simulink model "modelo_control_geoposicion"  (Simulink 7.5)
settings: Solver=ode45  StartTime=0.0  StopTime=10.0  RelTol=1e-3
settings Model: Creator=ARTURO  LastModifiedBy=ARTURO

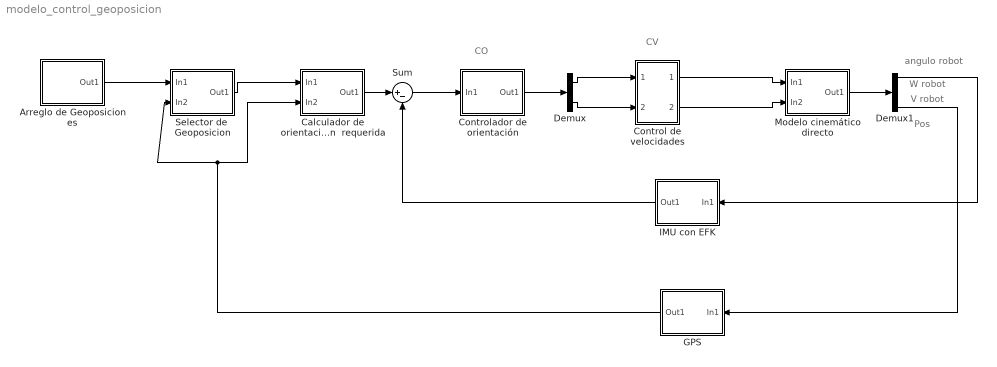
== system modelo_control_geoposicion ==
  note: W robot
  note: V robot
  note: angulo robot
  note: CV
  note: CO
  note: Pos
  Arreglo de Geoposiciones : Subsystem
  Calculador de orientación  requerida : Subsystem
  Control de velocidades : Subsystem
  Controlador de orientación : Subsystem
  Demux : Demux  Outputs=2
  Demux1 : Demux
  GPS : Subsystem
  IMU con EFK : Subsystem
  Modelo cinemático directo : Subsystem
  Selector de  Geoposicion : Subsystem
  Sum : Sum  Inputs=|+-  OutDataType=fixdt(1, 16)  OutScaling=2^0
  wires:
  Demux/1 -> Control de velocidades/1(In1)
  Demux/2 -> Control de velocidades/2(In2)
  Modelo cinemático directo/1(Out1) -> Demux1/1
  Control de velocidades/1(Out1) -> Modelo cinemático directo/1(In1)
  Control de velocidades/2(Out2) -> Modelo cinemático directo/2(In2)
  Calculador de orientación  requerida/1(Out1) -> Sum/1
  Sum/1 -> Controlador de orientación/1(In1)
  Controlador de orientación/1(Out1) -> Demux/1
  Demux1/1 -> IMU con EFK/1(In1)
  IMU con EFK/1(Out1) -> Sum/2
  Demux1/4 -> GPS/1(In1)
  Selector de  Geoposicion/1(Out1) -> Calculador de orientación  requerida/1(In1)
  GPS/1(Out1) -> Calculador de orientación  requerida/2(In2), Selector de  Geoposicion/2(In2)
  Arreglo de Geoposiciones/1(Out1) -> Selector de  Geoposicion/1(In1)

== system modelo_control_geoposicion/Arreglo de Geoposiciones ==
  Out1 : Outport  OutDataType=fixdt(1, 16)  OutScaling=2^0

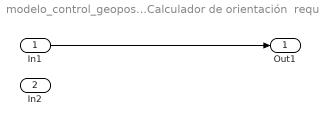
== system modelo_control_geoposicion/Calculador de orientación  requerida ==
  In1 : Inport  OutDataType=fixdt(1, 16)  OutScaling=2^0
  In2 : Inport  Port=2  OutDataType=fixdt(1, 16)  OutScaling=2^0
  Out1 : Outport  OutDataType=fixdt(1, 16)  OutScaling=2^0
  wires:
  In1/1 -> Out1/1

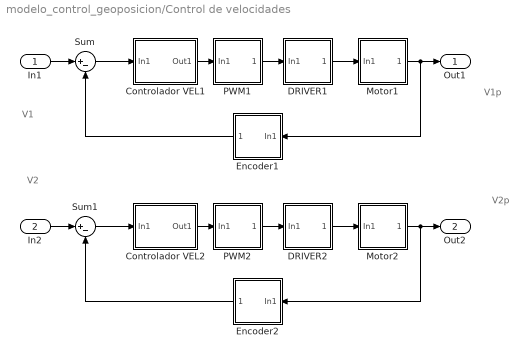
== system modelo_control_geoposicion/Control de velocidades ==
  note: V1
  note: V2
  note: V1p
  note: V2p
  In1 : Inport
  In2 : Inport  Port=2
  Controlador VEL1 : Subsystem
  Controlador VEL2 : Subsystem
  DRIVER1 : Subsystem
  DRIVER2 : Subsystem
  Encoder1 : Subsystem
  Encoder2 : Subsystem
  Motor1 : Subsystem
  Motor2 : Subsystem
  PWM1 : Subsystem
  PWM2 : Subsystem
  Sum : Sum  Inputs=|+-  OutDataType=fixdt(1, 16)  OutScaling=2^0
  Sum1 : Sum  Inputs=|+-  OutDataType=fixdt(1, 16)  OutScaling=2^0
  Out1 : Outport
  Out2 : Outport  Port=2
  wires:
  Sum/1 -> Controlador VEL1/1(In1)
  Controlador VEL1/1(Out1) -> PWM1/1(In1)
  PWM1/1(Out1) -> DRIVER1/1(In1)
  DRIVER1/1(Out1) -> Motor1/1(In1)
  Motor1/1(Out1) -> Encoder1/1(In1), Out1/1
  Encoder1/1(Out1) -> Sum/2
  Sum1/1 -> Controlador VEL2/1(In1)
  Controlador VEL2/1(Out1) -> PWM2/1(In1)
  PWM2/1(Out1) -> DRIVER2/1(In1)
  DRIVER2/1(Out1) -> Motor2/1(In1)
  Motor2/1(Out1) -> Encoder2/1(In1), Out2/1
  Encoder2/1(Out1) -> Sum1/2
  In1/1 -> Sum/1
  In2/1 -> Sum1/1

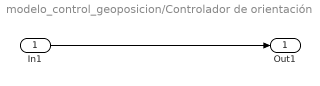
== system modelo_control_geoposicion/Controlador de orientación ==
  In1 : Inport  OutDataType=fixdt(1, 16)  OutScaling=2^0
  Out1 : Outport  OutDataType=fixdt(1, 16)  OutScaling=2^0
  wires:
  In1/1 -> Out1/1

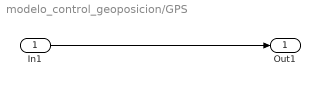
== system modelo_control_geoposicion/GPS ==
  In1 : Inport  OutDataType=fixdt(1, 16)  OutScaling=2^0
  Out1 : Outport  OutDataType=fixdt(1, 16)  OutScaling=2^0
  wires:
  In1/1 -> Out1/1

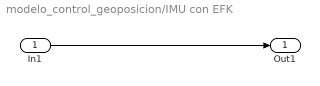
== system modelo_control_geoposicion/IMU con EFK ==
  In1 : Inport  OutDataType=fixdt(1, 16)  OutScaling=2^0
  Out1 : Outport  OutDataType=fixdt(1, 16)  OutScaling=2^0
  wires:
  In1/1 -> Out1/1

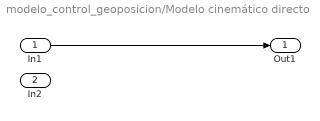
== system modelo_control_geoposicion/Modelo cinemático directo ==
  In1 : Inport  OutDataType=fixdt(1, 16)  OutScaling=2^0
  In2 : Inport  Port=2  OutDataType=fixdt(1, 16)  OutScaling=2^0
  Out1 : Outport  OutDataType=fixdt(1, 16)  OutScaling=2^0
  wires:
  In1/1 -> Out1/1

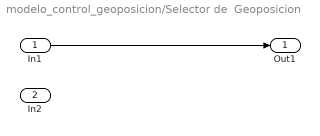
== system modelo_control_geoposicion/Selector de  Geoposicion ==
  In1 : Inport  OutDataType=fixdt(1, 16)  OutScaling=2^0
  In2 : Inport  Port=2  OutDataType=fixdt(1, 16)  OutScaling=2^0
  Out1 : Outport  OutDataType=fixdt(1, 16)  OutScaling=2^0
  wires:
  In1/1 -> Out1/1

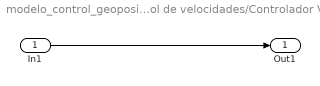
== system modelo_control_geoposicion/Control de velocidades/Controlador VEL1 ==
  In1 : Inport  OutDataType=fixdt(1, 16)  OutScaling=2^0
  Out1 : Outport  OutDataType=fixdt(1, 16)  OutScaling=2^0
  wires:
  In1/1 -> Out1/1

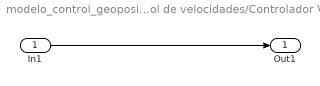
== system modelo_control_geoposicion/Control de velocidades/Controlador VEL2 ==
  In1 : Inport  OutDataType=fixdt(1, 16)  OutScaling=2^0
  Out1 : Outport  OutDataType=fixdt(1, 16)  OutScaling=2^0
  wires:
  In1/1 -> Out1/1

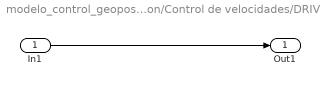
== system modelo_control_geoposicion/Control de velocidades/DRIVER1 ==
  In1 : Inport  OutDataType=fixdt(1, 16)  OutScaling=2^0
  Out1 : Outport  OutDataType=fixdt(1, 16)  OutScaling=2^0
  wires:
  In1/1 -> Out1/1

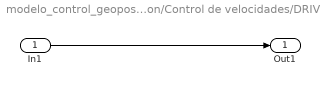
== system modelo_control_geoposicion/Control de velocidades/DRIVER2 ==
  In1 : Inport  OutDataType=fixdt(1, 16)  OutScaling=2^0
  Out1 : Outport  OutDataType=fixdt(1, 16)  OutScaling=2^0
  wires:
  In1/1 -> Out1/1

== system modelo_control_geoposicion/Control de velocidades/Encoder1 ==
  In1 : Inport  OutDataType=fixdt(1, 16)  OutScaling=2^0
  Out1 : Outport  OutDataType=fixdt(1, 16)  OutScaling=2^0
  wires:
  In1/1 -> Out1/1

== system modelo_control_geoposicion/Control de velocidades/Encoder2 ==
  In1 : Inport  OutDataType=fixdt(1, 16)  OutScaling=2^0
  Out1 : Outport  OutDataType=fixdt(1, 16)  OutScaling=2^0
  wires:
  In1/1 -> Out1/1

== system modelo_control_geoposicion/Control de velocidades/Motor1 ==
  In1 : Inport  OutDataType=fixdt(1, 16)  OutScaling=2^0
  Out1 : Outport  OutDataType=fixdt(1, 16)  OutScaling=2^0
  wires:
  In1/1 -> Out1/1

== system modelo_control_geoposicion/Control de velocidades/Motor2 ==
  In1 : Inport  OutDataType=fixdt(1, 16)  OutScaling=2^0
  Out1 : Outport  OutDataType=fixdt(1, 16)  OutScaling=2^0
  wires:
  In1/1 -> Out1/1

== system modelo_control_geoposicion/Control de velocidades/PWM1 ==
  In1 : Inport  OutDataType=fixdt(1, 16)  OutScaling=2^0
  Out1 : Outport  OutDataType=fixdt(1, 16)  OutScaling=2^0
  wires:
  In1/1 -> Out1/1

== system modelo_control_geoposicion/Control de velocidades/PWM2 ==
  In1 : Inport  OutDataType=fixdt(1, 16)  OutScaling=2^0
  Out1 : Outport  OutDataType=fixdt(1, 16)  OutScaling=2^0
  wires:
  In1/1 -> Out1/1
